simulink model "RoboticFish_NGC"  (R2023b)
settings: Solver=ode4  StartTime=0.0  StopTime=89  FixedStep=0.00025  RelTol=1e-3  EnableMultiTasking=on
undefined symbols (not defined in the file): Ref, uCMD
libraries: sharedutil x11, slpidlib x8, dspsigops x2, matrix_library x1, SignalEditorBlockLib x1, vrlib x1
(part 2 of 3)

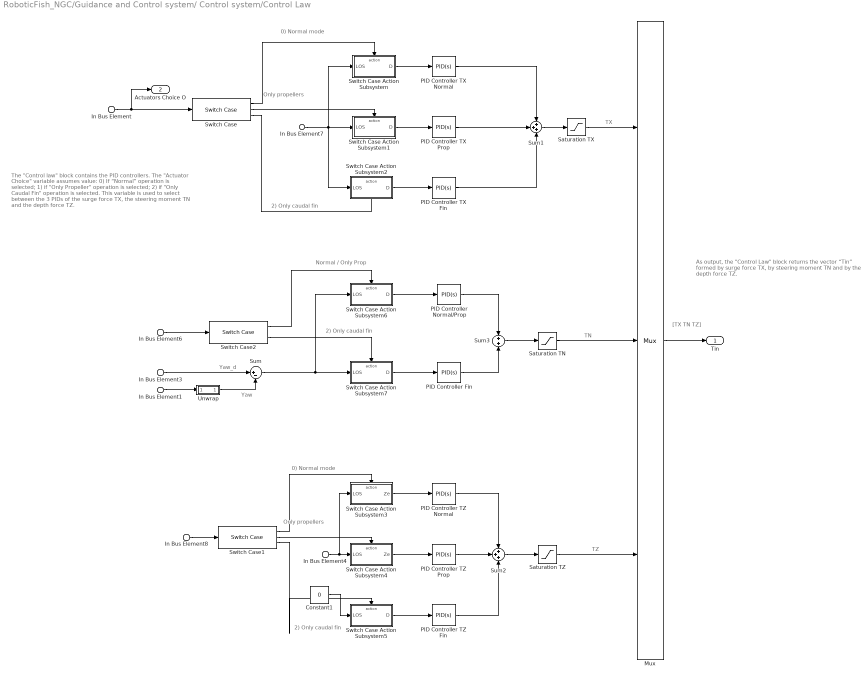
== system RoboticFish_NGC/Guidance and Control system/ Control system/Control Law ==
  note: Normal / Only Prop
  note: 2) Only caudal fin
  note: As output, the "Control Law" block returns the vector “Tin” formed by surge force TX, by steering moment TN and by the depth force TZ.
  note: The "Control law" block contains the PID controllers.
      | The "Actuator Choice" variable assumes value:
      | 0) If “Normal” operation is selected;
      | 1) if "Only Propeller" operation is selected;
      | 2) if "Only Caudal Fin" operation is selected.
      | This variable is used to select between the 3 PIDs of the surge force TX, the steering moment TN and the depth force TZ.
  note: [TX TN TZ]
  note: TZ
  note: TN
  note: TX
  note: 2) Only caudal fin
  note: Only propellers
  note: 0) Normal mode
  note: 0) Normal mode
  note: 2) Only caudal fin
  note: Only propellers
  note: Yaw
  note: Yaw_d
  In Bus Element7 : Inport  PortName=LOS  Element=D
  In Bus Element4 : Inport  PortName=LOS  Element=Ze
  In Bus Element3 : Inport  PortName=LOS  Element=Yaw_d
  In Bus Element : Inport  Port=2  PortName=P  Element=Actuators Choice
  In Bus Element8 : Inport  Port=2  PortName=P  Element=Actuators Choice
  In Bus Element6 : Inport  Port=2  PortName=P  Element=Actuators Choice
  In Bus Element1 : Inport  Port=3  PortName=Estimate States  Element=Position.Yaw
  Constant1 : Constant  Value=0
  Mux : Mux  Inputs=3
  PID Controller Fin : slpidlib/PID Controller  Controller=PID  Form=Parallel  TimeDomain=Continuous-time  UseExternalTs=off  SampleTime=-1  IntegratorMethod=Forward Euler  FilterMethod=Forward Euler  ControllerParametersSource=internal  P=0.1  I=0  UseKiTs=off  D=0.01  N=100  UseFilter=on  TunerSelectOption=Transfer Function Based (PID Tuner App)  InitialConditionSource=internal  InitialConditionForIntegrator=0  InitialConditionForFilter=0  DifferentiatorICPrevScaledInput=0  ExternalReset=none  TrackingMode=off  Kt=1  LimitOutput=off  SatLimitsSource=internal  UpperSaturationLimit=inf  LowerSaturationLimit=-inf  LinearizeAsGain=on  AntiWindupMode=none  Kb=1  LimitIntegrator=off  UpperIntegratorSaturationLimit=inf  LowerIntegratorSaturationLimit=-inf  POutMin=[]  POutMax=[]  IOutMin=[]  IOutMax=[]  DOutMin=[]  DOutMax=[]  NOutMin=[]  NOutMax=[]  SumOutMin=[]  SumOutMax=[]  SaturationOutMin=[]  SaturationOutMax=[]  PParamMin=[]  PParamMax=[]  IParamMin=[]  IParamMax=[]  DParamMin=[]  DParamMax=[]  NParamMin=[]  NParamMax=[]  KbParamMin=[]  KbParamMax=[]  KtParamMin=[]  KtParamMax=[]  KbOutMin=[]  KbOutMax=[]  KtOutMin=[]  KtOutMax=[]  IntegratorOutMin=[]  IntegratorOutMax=[]  FilterOutMin=[]  FilterOutMax=[]  SumI1OutMin=[]  SumI1OutMax=[]  SumI2OutMin=[]  SumI2OutMax=[]  SumI3OutMin=[]  SumI3OutMax=[]  SumI4OutMin=[]  SumI4OutMax=[]  SumDOutMin=[]  SumDOutMax=[]  DifferentiatorOutMin=[]  DifferentiatorOutMax=[]  FilterDiffOutCoefMin=[]  FilterDiffOutCoefMax=[]  ReciprocalOutMin=[]  ReciprocalOutMax=[]  SumDenOutMin=[]  SumDenOutMax=[]  SumNumOutMin=[]  SumNumOutMax=[]  DivideOutMin=[]  DivideOutMax=[]  UdiffTsProdOutMin=[]  UdiffTsProdOutMax=[]  NTsProdOutMin=[]  NTsProdOutMax=[]  UintegralTsProdOutMin=[]  UintegralTsProdOutMax=[]  UngainTsProdOutMin=[]  UngainTsProdOutMax=[]  ClampingZeroOutDataTypeStr=Inherit: Inherit via back propagation  ClampingZeroOutMin=[]  ClampingZeroOutMax=[]  FilterDenConstantOutDataTypeStr=Inherit: Inherit via back propagation  FilterDenConstantOutMin=[]  FilterDenConstantOutMax=[]  PCopyOutDataTypeStr=Inherit: Inherit via back propagation  PCopyOutMin=[]  PCopyOutMax=[]  NCopyOutDataTypeStr=Inherit: Inherit via back propagation  NCopyOutMin=[]  NCopyOutMax=[]  IntegratorContinuousStateAttributes=''  IntegratorStateMustResolveToSignalObject=off  IntegratorRTWStateStorageClass=Auto  FilterContinuousStateAttributes=''  FilterStateMustResolveToSignalObject=off  FilterRTWStateStorageClass=Auto  ParallelPVariant=InternalParameters  IdealPVariant=Disabled  IVariant=InternalParameters  DVariant=InternalParameters  IntegratorVariant=Continuous  SatVariant=Disabled  AWVariant=Passthrough  PCopyVariant=Disabled  TRVariant=Disabled  FdbkBlocksVariant=Forward  IdealPFdbkVariant=Disabled  SatFdbkVariant=Disabled  DerivativeFilterVariant=ContFilter  NVariant=InternalParameters  NCopyVariant=Disabled  FilterICVariant=InternalICsFilter  IntegratorICVariant=InternalICs  ExternalResetVariant=Disabled  TRSumVariant=Passthrough  SumFdbkVariant=Disabled  SumVariant=Sum_PID  TsampFilterVariant=InternalTs  TsampNgainVariant=Passthrough  TsampIntegralVariant=Disabled_SignalSpec  ExternalSaturationOutDataTypeStr=Inherit: Same as second input
  PID Controller Normal/Prop : slpidlib/PID Controller  Controller=PID  Form=Parallel  TimeDomain=Continuous-time  UseExternalTs=off  SampleTime=-1  IntegratorMethod=Forward Euler  FilterMethod=Forward Euler  ControllerParametersSource=internal  P=2  I=0  UseKiTs=off  D=1  N=100  UseFilter=on  TunerSelectOption=Transfer Function Based (PID Tuner App)  InitialConditionSource=internal  InitialConditionForIntegrator=0  InitialConditionForFilter=0  DifferentiatorICPrevScaledInput=0  ExternalReset=none  TrackingMode=off  Kt=1  LimitOutput=off  SatLimitsSource=internal  UpperSaturationLimit=inf  LowerSaturationLimit=-inf  LinearizeAsGain=on  AntiWindupMode=none  Kb=1  LimitIntegrator=off  UpperIntegratorSaturationLimit=inf  LowerIntegratorSaturationLimit=-inf  POutMin=[]  POutMax=[]  IOutMin=[]  IOutMax=[]  DOutMin=[]  DOutMax=[]  NOutMin=[]  NOutMax=[]  SumOutMin=[]  SumOutMax=[]  SaturationOutMin=[]  SaturationOutMax=[]  PParamMin=[]  PParamMax=[]  IParamMin=[]  IParamMax=[]  DParamMin=[]  DParamMax=[]  NParamMin=[]  NParamMax=[]  KbParamMin=[]  KbParamMax=[]  KtParamMin=[]  KtParamMax=[]  KbOutMin=[]  KbOutMax=[]  KtOutMin=[]  KtOutMax=[]  IntegratorOutMin=[]  IntegratorOutMax=[]  FilterOutMin=[]  FilterOutMax=[]  SumI1OutMin=[]  SumI1OutMax=[]  SumI2OutMin=[]  SumI2OutMax=[]  SumI3OutMin=[]  SumI3OutMax=[]  SumI4OutMin=[]  SumI4OutMax=[]  SumDOutMin=[]  SumDOutMax=[]  DifferentiatorOutMin=[]  DifferentiatorOutMax=[]  FilterDiffOutCoefMin=[]  FilterDiffOutCoefMax=[]  ReciprocalOutMin=[]  ReciprocalOutMax=[]  SumDenOutMin=[]  SumDenOutMax=[]  SumNumOutMin=[]  SumNumOutMax=[]  DivideOutMin=[]  DivideOutMax=[]  UdiffTsProdOutMin=[]  UdiffTsProdOutMax=[]  NTsProdOutMin=[]  NTsProdOutMax=[]  UintegralTsProdOutMin=[]  UintegralTsProdOutMax=[]  UngainTsProdOutMin=[]  UngainTsProdOutMax=[]  ClampingZeroOutDataTypeStr=Inherit: Inherit via back propagation  ClampingZeroOutMin=[]  ClampingZeroOutMax=[]  FilterDenConstantOutDataTypeStr=Inherit: Inherit via back propagation  FilterDenConstantOutMin=[]  FilterDenConstantOutMax=[]  PCopyOutDataTypeStr=Inherit: Inherit via back propagation  PCopyOutMin=[]  PCopyOutMax=[]  NCopyOutDataTypeStr=Inherit: Inherit via back propagation  NCopyOutMin=[]  NCopyOutMax=[]  IntegratorContinuousStateAttributes=''  IntegratorStateMustResolveToSignalObject=off  IntegratorRTWStateStorageClass=Auto  FilterContinuousStateAttributes=''  FilterStateMustResolveToSignalObject=off  FilterRTWStateStorageClass=Auto  ParallelPVariant=InternalParameters  IdealPVariant=Disabled  IVariant=InternalParameters  DVariant=InternalParameters  IntegratorVariant=Continuous  SatVariant=Disabled  AWVariant=Passthrough  PCopyVariant=Disabled  TRVariant=Disabled  FdbkBlocksVariant=Forward  IdealPFdbkVariant=Disabled  SatFdbkVariant=Disabled  DerivativeFilterVariant=ContFilter  NVariant=InternalParameters  NCopyVariant=Disabled  FilterICVariant=InternalICsFilter  IntegratorICVariant=InternalICs  ExternalResetVariant=Disabled  TRSumVariant=Passthrough  SumFdbkVariant=Disabled  SumVariant=Sum_PID  TsampFilterVariant=InternalTs  TsampNgainVariant=Passthrough  TsampIntegralVariant=Disabled_SignalSpec  ExternalSaturationOutDataTypeStr=Inherit: Same as second input
  PID Controller TX Fin : slpidlib/PID Controller  Controller=PID  Form=Parallel  TimeDomain=Continuous-time  UseExternalTs=off  SampleTime=-1  IntegratorMethod=Forward Euler  FilterMethod=Forward Euler  ControllerParametersSource=internal  P=1  I=0  UseKiTs=off  D=0  N=100  UseFilter=on  TunerSelectOption=Transfer Function Based (PID Tuner App)  InitialConditionSource=internal  InitialConditionForIntegrator=0  InitialConditionForFilter=0  DifferentiatorICPrevScaledInput=0  ExternalReset=none  TrackingMode=off  Kt=1  LimitOutput=off  SatLimitsSource=internal  UpperSaturationLimit=inf  LowerSaturationLimit=-inf  LinearizeAsGain=on  AntiWindupMode=none  Kb=1  LimitIntegrator=off  UpperIntegratorSaturationLimit=inf  LowerIntegratorSaturationLimit=-inf  POutMin=[]  POutMax=[]  IOutMin=[]  IOutMax=[]  DOutMin=[]  DOutMax=[]  NOutMin=[]  NOutMax=[]  SumOutMin=[]  SumOutMax=[]  SaturationOutMin=[]  SaturationOutMax=[]  PParamMin=[]  PParamMax=[]  IParamMin=[]  IParamMax=[]  DParamMin=[]  DParamMax=[]  NParamMin=[]  NParamMax=[]  KbParamMin=[]  KbParamMax=[]  KtParamMin=[]  KtParamMax=[]  KbOutMin=[]  KbOutMax=[]  KtOutMin=[]  KtOutMax=[]  IntegratorOutMin=[]  IntegratorOutMax=[]  FilterOutMin=[]  FilterOutMax=[]  SumI1OutMin=[]  SumI1OutMax=[]  SumI2OutMin=[]  SumI2OutMax=[]  SumI3OutMin=[]  SumI3OutMax=[]  SumI4OutMin=[]  SumI4OutMax=[]  SumDOutMin=[]  SumDOutMax=[]  DifferentiatorOutMin=[]  DifferentiatorOutMax=[]  FilterDiffOutCoefMin=[]  FilterDiffOutCoefMax=[]  ReciprocalOutMin=[]  ReciprocalOutMax=[]  SumDenOutMin=[]  SumDenOutMax=[]  SumNumOutMin=[]  SumNumOutMax=[]  DivideOutMin=[]  DivideOutMax=[]  UdiffTsProdOutMin=[]  UdiffTsProdOutMax=[]  NTsProdOutMin=[]  NTsProdOutMax=[]  UintegralTsProdOutMin=[]  UintegralTsProdOutMax=[]  UngainTsProdOutMin=[]  UngainTsProdOutMax=[]  ClampingZeroOutDataTypeStr=Inherit: Inherit via back propagation  ClampingZeroOutMin=[]  ClampingZeroOutMax=[]  FilterDenConstantOutDataTypeStr=Inherit: Inherit via back propagation  FilterDenConstantOutMin=[]  FilterDenConstantOutMax=[]  PCopyOutDataTypeStr=Inherit: Inherit via back propagation  PCopyOutMin=[]  PCopyOutMax=[]  NCopyOutDataTypeStr=Inherit: Inherit via back propagation  NCopyOutMin=[]  NCopyOutMax=[]  IntegratorContinuousStateAttributes=''  IntegratorStateMustResolveToSignalObject=off  IntegratorRTWStateStorageClass=Auto  FilterContinuousStateAttributes=''  FilterStateMustResolveToSignalObject=off  FilterRTWStateStorageClass=Auto  ParallelPVariant=InternalParameters  IdealPVariant=Disabled  IVariant=InternalParameters  DVariant=InternalParameters  IntegratorVariant=Continuous  SatVariant=Disabled  AWVariant=Passthrough  PCopyVariant=Disabled  TRVariant=Disabled  FdbkBlocksVariant=Forward  IdealPFdbkVariant=Disabled  SatFdbkVariant=Disabled  DerivativeFilterVariant=ContFilter  NVariant=InternalParameters  NCopyVariant=Disabled  FilterICVariant=InternalICsFilter  IntegratorICVariant=InternalICs  ExternalResetVariant=Disabled  TRSumVariant=Passthrough  SumFdbkVariant=Disabled  SumVariant=Sum_PID  TsampFilterVariant=InternalTs  TsampNgainVariant=Passthrough  TsampIntegralVariant=Disabled_SignalSpec  ExternalSaturationOutDataTypeStr=Inherit: Same as second input
  PID Controller TX Normal : slpidlib/PID Controller  Controller=PID  Form=Parallel  TimeDomain=Continuous-time  UseExternalTs=off  SampleTime=-1  IntegratorMethod=Forward Euler  FilterMethod=Forward Euler  ControllerParametersSource=internal  P=1  I=0  UseKiTs=off  D=0.2695  N=100  UseFilter=on  TunerSelectOption=Transfer Function Based (PID Tuner App)  InitialConditionSource=internal  InitialConditionForIntegrator=0  InitialConditionForFilter=0  DifferentiatorICPrevScaledInput=0  ExternalReset=none  TrackingMode=off  Kt=1  LimitOutput=off  SatLimitsSource=internal  UpperSaturationLimit=inf  LowerSaturationLimit=-inf  LinearizeAsGain=on  AntiWindupMode=none  Kb=1  LimitIntegrator=off  UpperIntegratorSaturationLimit=inf  LowerIntegratorSaturationLimit=-inf  POutMin=[]  POutMax=[]  IOutMin=[]  IOutMax=[]  DOutMin=[]  DOutMax=[]  NOutMin=[]  NOutMax=[]  SumOutMin=[]  SumOutMax=[]  SaturationOutMin=[]  SaturationOutMax=[]  PParamMin=[]  PParamMax=[]  IParamMin=[]  IParamMax=[]  DParamMin=[]  DParamMax=[]  NParamMin=[]  NParamMax=[]  KbParamMin=[]  KbParamMax=[]  KtParamMin=[]  KtParamMax=[]  KbOutMin=[]  KbOutMax=[]  KtOutMin=[]  KtOutMax=[]  IntegratorOutMin=[]  IntegratorOutMax=[]  FilterOutMin=[]  FilterOutMax=[]  SumI1OutMin=[]  SumI1OutMax=[]  SumI2OutMin=[]  SumI2OutMax=[]  SumI3OutMin=[]  SumI3OutMax=[]  SumI4OutMin=[]  SumI4OutMax=[]  SumDOutMin=[]  SumDOutMax=[]  DifferentiatorOutMin=[]  DifferentiatorOutMax=[]  FilterDiffOutCoefMin=[]  FilterDiffOutCoefMax=[]  ReciprocalOutMin=[]  ReciprocalOutMax=[]  SumDenOutMin=[]  SumDenOutMax=[]  SumNumOutMin=[]  SumNumOutMax=[]  DivideOutMin=[]  DivideOutMax=[]  UdiffTsProdOutMin=[]  UdiffTsProdOutMax=[]  NTsProdOutMin=[]  NTsProdOutMax=[]  UintegralTsProdOutMin=[]  UintegralTsProdOutMax=[]  UngainTsProdOutMin=[]  UngainTsProdOutMax=[]  ClampingZeroOutDataTypeStr=Inherit: Inherit via back propagation  ClampingZeroOutMin=[]  ClampingZeroOutMax=[]  FilterDenConstantOutDataTypeStr=Inherit: Inherit via back propagation  FilterDenConstantOutMin=[]  FilterDenConstantOutMax=[]  PCopyOutDataTypeStr=Inherit: Inherit via back propagation  PCopyOutMin=[]  PCopyOutMax=[]  NCopyOutDataTypeStr=Inherit: Inherit via back propagation  NCopyOutMin=[]  NCopyOutMax=[]  IntegratorContinuousStateAttributes=''  IntegratorStateMustResolveToSignalObject=off  IntegratorRTWStateStorageClass=Auto  FilterContinuousStateAttributes=''  FilterStateMustResolveToSignalObject=off  FilterRTWStateStorageClass=Auto  ParallelPVariant=InternalParameters  IdealPVariant=Disabled  IVariant=InternalParameters  DVariant=InternalParameters  IntegratorVariant=Continuous  SatVariant=Disabled  AWVariant=Passthrough  PCopyVariant=Disabled  TRVariant=Disabled  FdbkBlocksVariant=Forward  IdealPFdbkVariant=Disabled  SatFdbkVariant=Disabled  DerivativeFilterVariant=ContFilter  NVariant=InternalParameters  NCopyVariant=Disabled  FilterICVariant=InternalICsFilter  IntegratorICVariant=InternalICs  ExternalResetVariant=Disabled  TRSumVariant=Passthrough  SumFdbkVariant=Disabled  SumVariant=Sum_PID  TsampFilterVariant=InternalTs  TsampNgainVariant=Passthrough  TsampIntegralVariant=Disabled_SignalSpec  ExternalSaturationOutDataTypeStr=Inherit: Same as second input
  PID Controller TX Prop : slpidlib/PID Controller  Controller=PID  Form=Parallel  TimeDomain=Continuous-time  UseExternalTs=off  SampleTime=-1  IntegratorMethod=Forward Euler  FilterMethod=Forward Euler  ControllerParametersSource=internal  P=1  I=0  UseKiTs=off  D=1.2  N=100  UseFilter=on  TunerSelectOption=Frequency Response Based  InitialConditionSource=internal  InitialConditionForIntegrator=0  InitialConditionForFilter=0  DifferentiatorICPrevScaledInput=0  ExternalReset=none  TrackingMode=off  Kt=1  LimitOutput=off  SatLimitsSource=internal  UpperSaturationLimit=inf  LowerSaturationLimit=-inf  LinearizeAsGain=on  AntiWindupMode=none  Kb=1  LimitIntegrator=off  UpperIntegratorSaturationLimit=inf  LowerIntegratorSaturationLimit=-inf  POutMin=[]  POutMax=[]  IOutMin=[]  IOutMax=[]  DOutMin=[]  DOutMax=[]  NOutMin=[]  NOutMax=[]  SumOutMin=[]  SumOutMax=[]  SaturationOutMin=[]  SaturationOutMax=[]  PParamMin=[]  PParamMax=[]  IParamMin=[]  IParamMax=[]  DParamMin=[]  DParamMax=[]  NParamMin=[]  NParamMax=[]  KbParamMin=[]  KbParamMax=[]  KtParamMin=[]  KtParamMax=[]  KbOutMin=[]  KbOutMax=[]  KtOutMin=[]  KtOutMax=[]  IntegratorOutMin=[]  IntegratorOutMax=[]  FilterOutMin=[]  FilterOutMax=[]  SumI1OutMin=[]  SumI1OutMax=[]  SumI2OutMin=[]  SumI2OutMax=[]  SumI3OutMin=[]  SumI3OutMax=[]  SumI4OutMin=[]  SumI4OutMax=[]  SumDOutMin=[]  SumDOutMax=[]  DifferentiatorOutMin=[]  DifferentiatorOutMax=[]  FilterDiffOutCoefMin=[]  FilterDiffOutCoefMax=[]  ReciprocalOutMin=[]  ReciprocalOutMax=[]  SumDenOutMin=[]  SumDenOutMax=[]  SumNumOutMin=[]  SumNumOutMax=[]  DivideOutMin=[]  DivideOutMax=[]  UdiffTsProdOutMin=[]  UdiffTsProdOutMax=[]  NTsProdOutMin=[]  NTsProdOutMax=[]  UintegralTsProdOutMin=[]  UintegralTsProdOutMax=[]  UngainTsProdOutMin=[]  UngainTsProdOutMax=[]  ClampingZeroOutDataTypeStr=Inherit: Inherit via back propagation  ClampingZeroOutMin=[]  ClampingZeroOutMax=[]  FilterDenConstantOutDataTypeStr=Inherit: Inherit via back propagation  FilterDenConstantOutMin=[]  FilterDenConstantOutMax=[]  PCopyOutDataTypeStr=Inherit: Inherit via back propagation  PCopyOutMin=[]  PCopyOutMax=[]  NCopyOutDataTypeStr=Inherit: Inherit via back propagation  NCopyOutMin=[]  NCopyOutMax=[]  IntegratorContinuousStateAttributes=''  IntegratorStateMustResolveToSignalObject=off  IntegratorRTWStateStorageClass=Auto  FilterContinuousStateAttributes=''  FilterStateMustResolveToSignalObject=off  FilterRTWStateStorageClass=Auto  ParallelPVariant=InternalParameters  IdealPVariant=Disabled  IVariant=InternalParameters  DVariant=InternalParameters  IntegratorVariant=Continuous  SatVariant=Disabled  AWVariant=Passthrough  PCopyVariant=Disabled  TRVariant=Disabled  FdbkBlocksVariant=Forward  IdealPFdbkVariant=Disabled  SatFdbkVariant=Disabled  DerivativeFilterVariant=ContFilter  NVariant=InternalParameters  NCopyVariant=Disabled  FilterICVariant=InternalICsFilter  IntegratorICVariant=InternalICs  ExternalResetVariant=Disabled  TRSumVariant=Passthrough  SumFdbkVariant=Disabled  SumVariant=Sum_PID  TsampFilterVariant=InternalTs  TsampNgainVariant=Passthrough  TsampIntegralVariant=Disabled_SignalSpec  ExternalSaturationOutDataTypeStr=Inherit: Same as second input
  PID Controller TZ Fin : slpidlib/PID Controller  Controller=PID  Form=Parallel  TimeDomain=Continuous-time  UseExternalTs=off  SampleTime=-1  IntegratorMethod=Forward Euler  FilterMethod=Forward Euler  ControllerParametersSource=internal  P=0.6  I=0  UseKiTs=off  D=0.6  N=100  UseFilter=on  TunerSelectOption=Transfer Function Based (PID Tuner App)  InitialConditionSource=internal  InitialConditionForIntegrator=0  InitialConditionForFilter=0  DifferentiatorICPrevScaledInput=0  ExternalReset=none  TrackingMode=off  Kt=1  LimitOutput=off  SatLimitsSource=internal  UpperSaturationLimit=inf  LowerSaturationLimit=-inf  LinearizeAsGain=on  AntiWindupMode=none  Kb=1  LimitIntegrator=off  UpperIntegratorSaturationLimit=inf  LowerIntegratorSaturationLimit=-inf  POutMin=[]  POutMax=[]  IOutMin=[]  IOutMax=[]  DOutMin=[]  DOutMax=[]  NOutMin=[]  NOutMax=[]  SumOutMin=[]  SumOutMax=[]  SaturationOutMin=[]  SaturationOutMax=[]  PParamMin=[]  PParamMax=[]  IParamMin=[]  IParamMax=[]  DParamMin=[]  DParamMax=[]  NParamMin=[]  NParamMax=[]  KbParamMin=[]  KbParamMax=[]  KtParamMin=[]  KtParamMax=[]  KbOutMin=[]  KbOutMax=[]  KtOutMin=[]  KtOutMax=[]  IntegratorOutMin=[]  IntegratorOutMax=[]  FilterOutMin=[]  FilterOutMax=[]  SumI1OutMin=[]  SumI1OutMax=[]  SumI2OutMin=[]  SumI2OutMax=[]  SumI3OutMin=[]  SumI3OutMax=[]  SumI4OutMin=[]  SumI4OutMax=[]  SumDOutMin=[]  SumDOutMax=[]  DifferentiatorOutMin=[]  DifferentiatorOutMax=[]  FilterDiffOutCoefMin=[]  FilterDiffOutCoefMax=[]  ReciprocalOutMin=[]  ReciprocalOutMax=[]  SumDenOutMin=[]  SumDenOutMax=[]  SumNumOutMin=[]  SumNumOutMax=[]  DivideOutMin=[]  DivideOutMax=[]  UdiffTsProdOutMin=[]  UdiffTsProdOutMax=[]  NTsProdOutMin=[]  NTsProdOutMax=[]  UintegralTsProdOutMin=[]  UintegralTsProdOutMax=[]  UngainTsProdOutMin=[]  UngainTsProdOutMax=[]  ClampingZeroOutDataTypeStr=Inherit: Inherit via back propagation  ClampingZeroOutMin=[]  ClampingZeroOutMax=[]  FilterDenConstantOutDataTypeStr=Inherit: Inherit via back propagation  FilterDenConstantOutMin=[]  FilterDenConstantOutMax=[]  PCopyOutDataTypeStr=Inherit: Inherit via back propagation  PCopyOutMin=[]  PCopyOutMax=[]  NCopyOutDataTypeStr=Inherit: Inherit via back propagation  NCopyOutMin=[]  NCopyOutMax=[]  IntegratorContinuousStateAttributes=''  IntegratorStateMustResolveToSignalObject=off  IntegratorRTWStateStorageClass=Auto  FilterContinuousStateAttributes=''  FilterStateMustResolveToSignalObject=off  FilterRTWStateStorageClass=Auto  ParallelPVariant=InternalParameters  IdealPVariant=Disabled  IVariant=InternalParameters  DVariant=InternalParameters  IntegratorVariant=Continuous  SatVariant=Disabled  AWVariant=Passthrough  PCopyVariant=Disabled  TRVariant=Disabled  FdbkBlocksVariant=Forward  IdealPFdbkVariant=Disabled  SatFdbkVariant=Disabled  DerivativeFilterVariant=ContFilter  NVariant=InternalParameters  NCopyVariant=Disabled  FilterICVariant=InternalICsFilter  IntegratorICVariant=InternalICs  ExternalResetVariant=Disabled  TRSumVariant=Passthrough  SumFdbkVariant=Disabled  SumVariant=Sum_PID  TsampFilterVariant=InternalTs  TsampNgainVariant=Passthrough  TsampIntegralVariant=Disabled_SignalSpec  ExternalSaturationOutDataTypeStr=Inherit: Same as second input
  PID Controller TZ Normal : slpidlib/PID Controller  Controller=PID  Form=Parallel  TimeDomain=Continuous-time  UseExternalTs=off  SampleTime=-1  IntegratorMethod=Forward Euler  FilterMethod=Forward Euler  ControllerParametersSource=internal  P=0.6  I=0  UseKiTs=off  D=0.6  N=100  UseFilter=on  TunerSelectOption=Transfer Function Based (PID Tuner App)  InitialConditionSource=internal  InitialConditionForIntegrator=0  InitialConditionForFilter=0  DifferentiatorICPrevScaledInput=0  ExternalReset=none  TrackingMode=off  Kt=1  LimitOutput=off  SatLimitsSource=internal  UpperSaturationLimit=inf  LowerSaturationLimit=-inf  LinearizeAsGain=on  AntiWindupMode=none  Kb=1  LimitIntegrator=off  UpperIntegratorSaturationLimit=inf  LowerIntegratorSaturationLimit=-inf  POutMin=[]  POutMax=[]  IOutMin=[]  IOutMax=[]  DOutMin=[]  DOutMax=[]  NOutMin=[]  NOutMax=[]  SumOutMin=[]  SumOutMax=[]  SaturationOutMin=[]  SaturationOutMax=[]  PParamMin=[]  PParamMax=[]  IParamMin=[]  IParamMax=[]  DParamMin=[]  DParamMax=[]  NParamMin=[]  NParamMax=[]  KbParamMin=[]  KbParamMax=[]  KtParamMin=[]  KtParamMax=[]  KbOutMin=[]  KbOutMax=[]  KtOutMin=[]  KtOutMax=[]  IntegratorOutMin=[]  IntegratorOutMax=[]  FilterOutMin=[]  FilterOutMax=[]  SumI1OutMin=[]  SumI1OutMax=[]  SumI2OutMin=[]  SumI2OutMax=[]  SumI3OutMin=[]  SumI3OutMax=[]  SumI4OutMin=[]  SumI4OutMax=[]  SumDOutMin=[]  SumDOutMax=[]  DifferentiatorOutMin=[]  DifferentiatorOutMax=[]  FilterDiffOutCoefMin=[]  FilterDiffOutCoefMax=[]  ReciprocalOutMin=[]  ReciprocalOutMax=[]  SumDenOutMin=[]  SumDenOutMax=[]  SumNumOutMin=[]  SumNumOutMax=[]  DivideOutMin=[]  DivideOutMax=[]  UdiffTsProdOutMin=[]  UdiffTsProdOutMax=[]  NTsProdOutMin=[]  NTsProdOutMax=[]  UintegralTsProdOutMin=[]  UintegralTsProdOutMax=[]  UngainTsProdOutMin=[]  UngainTsProdOutMax=[]  ClampingZeroOutDataTypeStr=Inherit: Inherit via back propagation  ClampingZeroOutMin=[]  ClampingZeroOutMax=[]  FilterDenConstantOutDataTypeStr=Inherit: Inherit via back propagation  FilterDenConstantOutMin=[]  FilterDenConstantOutMax=[]  PCopyOutDataTypeStr=Inherit: Inherit via back propagation  PCopyOutMin=[]  PCopyOutMax=[]  NCopyOutDataTypeStr=Inherit: Inherit via back propagation  NCopyOutMin=[]  NCopyOutMax=[]  IntegratorContinuousStateAttributes=''  IntegratorStateMustResolveToSignalObject=off  IntegratorRTWStateStorageClass=Auto  FilterContinuousStateAttributes=''  FilterStateMustResolveToSignalObject=off  FilterRTWStateStorageClass=Auto  ParallelPVariant=InternalParameters  IdealPVariant=Disabled  IVariant=InternalParameters  DVariant=InternalParameters  IntegratorVariant=Continuous  SatVariant=Disabled  AWVariant=Passthrough  PCopyVariant=Disabled  TRVariant=Disabled  FdbkBlocksVariant=Forward  IdealPFdbkVariant=Disabled  SatFdbkVariant=Disabled  DerivativeFilterVariant=ContFilter  NVariant=InternalParameters  NCopyVariant=Disabled  FilterICVariant=InternalICsFilter  IntegratorICVariant=InternalICs  ExternalResetVariant=Disabled  TRSumVariant=Passthrough  SumFdbkVariant=Disabled  SumVariant=Sum_PID  TsampFilterVariant=InternalTs  TsampNgainVariant=Passthrough  TsampIntegralVariant=Disabled_SignalSpec  ExternalSaturationOutDataTypeStr=Inherit: Same as second input
  PID Controller TZ Prop : slpidlib/PID Controller  Controller=PID  Form=Parallel  TimeDomain=Continuous-time  UseExternalTs=off  SampleTime=-1  IntegratorMethod=Forward Euler  FilterMethod=Forward Euler  ControllerParametersSource=internal  P=0.2  I=0  UseKiTs=off  D=0.2  N=100  UseFilter=on  TunerSelectOption=Transfer Function Based (PID Tuner App)  InitialConditionSource=internal  InitialConditionForIntegrator=0  InitialConditionForFilter=0  DifferentiatorICPrevScaledInput=0  ExternalReset=none  TrackingMode=off  Kt=1  LimitOutput=off  SatLimitsSource=internal  UpperSaturationLimit=inf  LowerSaturationLimit=-inf  LinearizeAsGain=on  AntiWindupMode=none  Kb=1  LimitIntegrator=off  UpperIntegratorSaturationLimit=inf  LowerIntegratorSaturationLimit=-inf  POutMin=[]  POutMax=[]  IOutMin=[]  IOutMax=[]  DOutMin=[]  DOutMax=[]  NOutMin=[]  NOutMax=[]  SumOutMin=[]  SumOutMax=[]  SaturationOutMin=[]  SaturationOutMax=[]  PParamMin=[]  PParamMax=[]  IParamMin=[]  IParamMax=[]  DParamMin=[]  DParamMax=[]  NParamMin=[]  NParamMax=[]  KbParamMin=[]  KbParamMax=[]  KtParamMin=[]  KtParamMax=[]  KbOutMin=[]  KbOutMax=[]  KtOutMin=[]  KtOutMax=[]  IntegratorOutMin=[]  IntegratorOutMax=[]  FilterOutMin=[]  FilterOutMax=[]  SumI1OutMin=[]  SumI1OutMax=[]  SumI2OutMin=[]  SumI2OutMax=[]  SumI3OutMin=[]  SumI3OutMax=[]  SumI4OutMin=[]  SumI4OutMax=[]  SumDOutMin=[]  SumDOutMax=[]  DifferentiatorOutMin=[]  DifferentiatorOutMax=[]  FilterDiffOutCoefMin=[]  FilterDiffOutCoefMax=[]  ReciprocalOutMin=[]  ReciprocalOutMax=[]  SumDenOutMin=[]  SumDenOutMax=[]  SumNumOutMin=[]  SumNumOutMax=[]  DivideOutMin=[]  DivideOutMax=[]  UdiffTsProdOutMin=[]  UdiffTsProdOutMax=[]  NTsProdOutMin=[]  NTsProdOutMax=[]  UintegralTsProdOutMin=[]  UintegralTsProdOutMax=[]  UngainTsProdOutMin=[]  UngainTsProdOutMax=[]  ClampingZeroOutDataTypeStr=Inherit: Inherit via back propagation  ClampingZeroOutMin=[]  ClampingZeroOutMax=[]  FilterDenConstantOutDataTypeStr=Inherit: Inherit via back propagation  FilterDenConstantOutMin=[]  FilterDenConstantOutMax=[]  PCopyOutDataTypeStr=Inherit: Inherit via back propagation  PCopyOutMin=[]  PCopyOutMax=[]  NCopyOutDataTypeStr=Inherit: Inherit via back propagation  NCopyOutMin=[]  NCopyOutMax=[]  IntegratorContinuousStateAttributes=''  IntegratorStateMustResolveToSignalObject=off  IntegratorRTWStateStorageClass=Auto  FilterContinuousStateAttributes=''  FilterStateMustResolveToSignalObject=off  FilterRTWStateStorageClass=Auto  ParallelPVariant=InternalParameters  IdealPVariant=Disabled  IVariant=InternalParameters  DVariant=InternalParameters  IntegratorVariant=Continuous  SatVariant=Disabled  AWVariant=Passthrough  PCopyVariant=Disabled  TRVariant=Disabled  FdbkBlocksVariant=Forward  IdealPFdbkVariant=Disabled  SatFdbkVariant=Disabled  DerivativeFilterVariant=ContFilter  NVariant=InternalParameters  NCopyVariant=Disabled  FilterICVariant=InternalICsFilter  IntegratorICVariant=InternalICs  ExternalResetVariant=Disabled  TRSumVariant=Passthrough  SumFdbkVariant=Disabled  SumVariant=Sum_PID  TsampFilterVariant=InternalTs  TsampNgainVariant=Passthrough  TsampIntegralVariant=Disabled_SignalSpec  ExternalSaturationOutDataTypeStr=Inherit: Same as second input
  Saturation TN : Saturate  UpperLimit=1.3090  LowerLimit=-1.3090
  Saturation TX : Saturate  UpperLimit=4  LowerLimit=0
  Saturation TZ : Saturate  UpperLimit=1  LowerLimit=-1
  Sum : Sum  Inputs=|+-
  Sum1 : Sum  Inputs=+++
  Sum2 : Sum  Inputs=+++
  Sum3 : Sum
  Switch Case : SwitchCase  CaseConditions={0,1,2}  ShowDefaultCase=off
  Switch Case Action Subsystem : Subsystem  TreatAsAtomicUnit=on
  Switch Case Action Subsystem1 : Subsystem  TreatAsAtomicUnit=on
  Switch Case Action Subsystem2 : Subsystem  TreatAsAtomicUnit=on
  Switch Case Action Subsystem3 : Subsystem  TreatAsAtomicUnit=on
  Switch Case Action Subsystem4 : Subsystem  TreatAsAtomicUnit=on
  Switch Case Action Subsystem5 : Subsystem  TreatAsAtomicUnit=on
  Switch Case Action Subsystem6 : Subsystem  TreatAsAtomicUnit=on
  Switch Case Action Subsystem7 : Subsystem  TreatAsAtomicUnit=on
  Switch Case1 : SwitchCase  CaseConditions={0,1,2}  ShowDefaultCase=off
  Switch Case2 : SwitchCase  CaseConditions={[0,1],2}  ShowDefaultCase=off
  Unwrap : Subsystem
  Tin : Outport  VectorParamsAs1DForOutWhenUnconnected=off
  Actuators Choice O : Outport  Port=2  VectorParamsAs1DForOutWhenUnconnected=off
  wires:
  In Bus Element/1 -> Switch Case/1, Actuators Choice O/1
  Switch Case/1 -> Switch Case Action Subsystem/Action
  Switch Case/2 -> Switch Case Action Subsystem1/Action
  Switch Case/3 -> Switch Case Action Subsystem2/Action
  In Bus Element7/1 -> Switch Case Action Subsystem1/1(LOS), Switch Case Action Subsystem/1(LOS), Switch Case Action Subsystem2/1(LOS)
  Switch Case Action Subsystem/1(D) -> PID Controller TX Normal/1
  Switch Case Action Subsystem1/1(D) -> PID Controller TX Prop/1
  Switch Case Action Subsystem2/1(D) -> PID Controller TX Fin/1
  PID Controller TX Prop/1 -> Sum1/2
  PID Controller TX Normal/1 -> Sum1/1
  Sum1/1 -> Saturation TX/1
  Sum2/1 -> Saturation TZ/1
  Switch Case Action Subsystem3/1(Ze) -> PID Controller TZ Normal/1
  Switch Case Action Subsystem5/1(D) -> PID Controller TZ Fin/1
  PID Controller TZ Prop/1 -> Sum2/2
  Switch Case Action Subsystem4/1(Ze) -> PID Controller TZ Prop/1
  Switch Case1/3 -> Switch Case Action Subsystem5/Action
  Switch Case1/2 -> Switch Case Action Subsystem4/Action
  Switch Case1/1 -> Switch Case Action Subsystem3/Action
  In Bus Element8/1 -> Switch Case1/1
  In Bus Element4/1 -> Switch Case Action Subsystem3/1(LOS), Switch Case Action Subsystem4/1(LOS)
  PID Controller TZ Fin/1 -> Sum2/3
  PID Controller TZ Normal/1 -> Sum2/1
  Constant1/1 -> Switch Case Action Subsystem5/1(LOS)
  Saturation TX/1 -> Mux/1
  Saturation TN/1 -> Mux/2
  Saturation TZ/1 -> Mux/3
  Mux/1 -> Tin/1
  Sum3/1 -> Saturation TN/1
  In Bus Element3/1 -> Sum/1
  In Bus Element1/1 -> Unwrap/1(yaw in)
  Unwrap/1(yaw out) -> Sum/2
  Switch Case2/1 -> Switch Case Action Subsystem6/Action
  Switch Case2/2 -> Switch Case Action Subsystem7/Action
  Switch Case Action Subsystem6/1(D) -> PID Controller Normal/Prop/1
  Switch Case Action Subsystem7/1(D) -> PID Controller Fin/1
  PID Controller Normal/Prop/1 -> Sum3/1
  PID Controller Fin/1 -> Sum3/2
  In Bus Element6/1 -> Switch Case2/1
  Sum/1 -> Switch Case Action Subsystem7/1(LOS), Switch Case Action Subsystem6/1(LOS)
  PID Controller TX Fin/1 -> Sum1/3

== system RoboticFish_NGC/Guidance and Control system/ Guidance system/Distance ==
  "[Xe Ye]" : Inport
  Demux : Demux  Outputs=2
  Plus : Sum
  Sqrt : Sqrt
  Square : Math  Operator=square  SignedPower=on
  Square1 : Math  Operator=square  SignedPower=on
  D : Outport  VectorParamsAs1DForOutWhenUnconnected=off
  wires:
  Demux/2 -> Square1/1  "Y"
  Square/1 -> Plus/1  "X^2"
  Square1/1 -> Plus/2  "Y^2"
  Plus/1 -> Sqrt/1  "X^2 + Y^2"
  Sqrt/1 -> D/1  "sqrt(X^2 + Y^2 )"
  Demux/1 -> Square/1  "X"
  "[Xe Ye]"/1 -> Demux/1

== system RoboticFish_NGC/Guidance and Control system/ Guidance system/LOS law ==
  note: To calculate the angle Yaw_d, the Unwrap Simulink block unwraps the input by adding or subtracting appropriate multiples of 𝜋 to remove phase discontinuities.
  "[Xe Ye]" : Inport
  Atan2 : Trigonometry  Operator=atan2
  Gain3 : Gain  Gain=180/pi
  Selector : Selector  InputPortWidth=2  IndexOptions=Index vector (dialog)  Indices=[2]  OutputSizes=1
  Selector3 : Selector  InputPortWidth=2  IndexOptions=Index vector (dialog)  Indices=[1]  OutputSizes=1
  "Unwrap " : dspsigops/Unwrap  tol=pi  InputProcessing=Columns as channels (frame based)  running=off
  Yaw_d : Outport  VectorParamsAs1DForOutWhenUnconnected=off
  wires:
  Selector/1 -> Atan2/1  "Ye"
  Selector3/1 -> Atan2/2  "Xe"
  "[Xe Ye]"/1 -> Selector3/1, Selector/1
  Gain3/1 -> Yaw_d/1
  Atan2/1 -> "Unwrap "/1
  "Unwrap "/1 -> Gain3/1

== system RoboticFish_NGC/Robotic-Fish Model & PropulsionSystem/Propulsion System/Horizontal Force and Moment (Tau_H) ==
  note: calcolo modulo: U=modulo(u v w)
  uHT3 : Inport
  uHT1 : Inport  Port=2
  uHT2 : Inport  Port=3
  nu_B : Inport  Port=4
  Dot Product : DotProduct  OutDataTypeStr=Inherit: Inherit via internal rule
  HT_prop : Constant  Value=HT_prop
  Matrix Multiply : Product  Multiplication=Matrix(*)
  Mux : Mux  Inputs=3
  Mux1 : Mux  Inputs=2
  Selector : Selector  InputPortWidth=6  IndexOptions=Index vector (dialog)  Indices=[1 2 3]  OutputSizes=1
  Sqrt : Sqrt
  Sum : Sum  Inputs=|++
  Tau_HT3 (Tau_Caudal_Fin) : Subsystem
  t : Clock
  Horizontal _Tau : Outport  VectorParamsAs1DForOutWhenUnconnected=off
  wires:
  uHT1/1 -> Mux1/1
  Tau_HT3 (Tau_Caudal_Fin)/1(Tau_HT3) -> Sum/1  "[Tau_surge_HT3 Tau_sway_HT3 0 0 0 Tau_yaw_HT3]"
  uHT2/1 -> Mux1/2
  Matrix Multiply/1 -> Sum/2  "[surge_HT1&HT2 0 0 0 0 yaw_HT1&HT2]"
  Mux1/1 -> Matrix Multiply/2
  HT_prop/1 -> Matrix Multiply/1
  Sum/1 -> Horizontal _Tau/1  "Tau_HT3+Tau_HT1&HT2"
  nu_B/1 -> Selector/1
  Selector/1 -> Dot Product/1, Dot Product/2
  Mux/1 -> Tau_HT3 (Tau_Caudal_Fin)/1("[U uHT3 t]")
  t/1 -> Mux/3
  Dot Product/1 -> Sqrt/1
  uHT3/1 -> Mux/2  "[f_%  Thetastr_%]"
  Sqrt/1 -> Mux/1  "U"

== system RoboticFish_NGC/Robotic-Fish Model & PropulsionSystem/Propulsion System/Subsystem ==
  D_uVT2  D_uVT3 : Inport
  uCMD : Inport  Port=2
  Bus Creator : BusCreator  Inputs=7
  Bus Selector : BusSelector  OutputSignals=D_VT2,D_VT3
  Bus Selector1 : BusSelector  OutputSignals=f_HT3,Thetastr_HT3,uHT1,uHT2,uVT1
  "ucmd " : Outport  VectorParamsAs1DForOutWhenUnconnected=off
  wires:
  D_uVT2  D_uVT3/1 -> Bus Selector/1
  uCMD/1 -> Bus Selector1/1
  Bus Selector/1 -> Bus Creator/6  "<D_VT2>"
  Bus Selector/2 -> Bus Creator/7  "<D_VT3>"
  Bus Selector1/5 -> Bus Creator/5  "<uVT1>"
  Bus Selector1/4 -> Bus Creator/4  "<uHT2>"
  Bus Selector1/3 -> Bus Creator/3  "<uHT1>"
  Bus Selector1/2 -> Bus Creator/2  "<Thetastr_HT3>"
  Bus Selector1/1 -> Bus Creator/1  "<f_HT3>"
  Bus Creator/1 -> "ucmd "/1

== system RoboticFish_NGC/Robotic-Fish Model & PropulsionSystem/Propulsion System/Vertical Force and Moment (Tau_V) ==
  note: Tau_VT2&VT3= [ 0 Ys Zs Ks Ms Ns ]
  note: Tau_VT1=[0 0 0 0 0 Fvt1]
  nu_B : Inport
  uVT1 : Inport  Port=2
  "[uVT2 uVT3]" : Inport  Port=3
  Bus Creator : BusCreator  Inputs=2
  Bus Selector : BusSelector  OutputSignals=uVT2,uVT3
  Constant : Constant  Value=VT_prop
  Matrix Multiply : Product  Multiplication=Matrix(*)
  Sum : Sum  Inputs=|++
  Tau_VT2&VT3 (Pectoral Fin) : Subsystem
  Vertical_Tau : Outport  VectorParamsAs1DForOutWhenUnconnected=off
  "[Delta_VT2 Delta_VT3]" : Outport  Port=2  VectorParamsAs1DForOutWhenUnconnected=off
  wires:
  nu_B/1 -> Tau_VT2&VT3 (Pectoral Fin)/3(nu_B)
  Constant/1 -> Matrix Multiply/1
  uVT1/1 -> Matrix Multiply/2
  Matrix Multiply/1 -> Sum/2
  Sum/1 -> Vertical_Tau/1
  Tau_VT2&VT3 (Pectoral Fin)/2(Delta_VT2) -> Bus Creator/1  "D_VT2"
  Tau_VT2&VT3 (Pectoral Fin)/3(Delta_VT3) -> Bus Creator/2  "D_VT3"
  Bus Creator/1 -> "[Delta_VT2 Delta_VT3]"/1
  Tau_VT2&VT3 (Pectoral Fin)/1("tau_VT2 & tau_VT3 ") -> Sum/1
  "[uVT2 uVT3]"/1 -> Bus Selector/1
  Bus Selector/1 -> Tau_VT2&VT3 (Pectoral Fin)/1("uVT2 ")  "<uVT2>"
  Bus Selector/2 -> Tau_VT2&VT3 (Pectoral Fin)/2(uVT3)  "<uVT3>"

== system RoboticFish_NGC/Robotic-Fish Model & PropulsionSystem/RF Dynamics and Kinematics (Attitude rappresentation: Quaternions)/6 DOF transformation ==
  note: p q r
  note: u v w
  note: e=[eta;e1;e2;e3]
  note: eta1dot
  note: eta2dot
  eta_E : Inport
  nu : Inport  Port=2
  E1(e) : Subsystem
  E2(e) : Subsystem
  Mux : Mux  Inputs=2
  Product : Product  Inputs=**  Multiplication=Matrix(*)  SaturateOnIntegerOverflow=on  OutDataTypeStr=Inherit: Same as first input
  Product1 : Product  Inputs=**  Multiplication=Matrix(*)  SaturateOnIntegerOverflow=on  OutDataTypeStr=Inherit: Same as first input
  Selector : Selector  InputPortWidth=7  IndexOptions=Index vector (dialog)  Indices=[4 5 6 7]  OutputSizes=1
  Selector1 : Selector  InputPortWidth=6  IndexOptions=Index vector (dialog)  Indices=[1 2 3]  OutputSizes=1
  Selector2 : Selector  InputPortWidth=6  IndexOptions=Index vector (dialog)  Indices=[4 5 6]  OutputSizes=1
  etadot = J(eta_E)*nu : Outport  VectorParamsAs1DForOutWhenUnconnected=off
  E1 : Outport  Port=2  VectorParamsAs1DForOutWhenUnconnected=off
  wires:
  Product1/1 -> Mux/2
  Mux/1 -> etadot = J(eta_E)*nu/1
  Product/1 -> Mux/1
  E2(e)/1(E2) -> Product1/1
  Selector2/1 -> Product1/2
  Selector1/1 -> Product/2
  nu/1 -> Selector2/1, Selector1/1
  E1(e)/1(E1) -> Product/1, E1/1
  eta_E/1 -> Selector/1
  Selector/1 -> E1(e)/1(e), E2(e)/1(e)

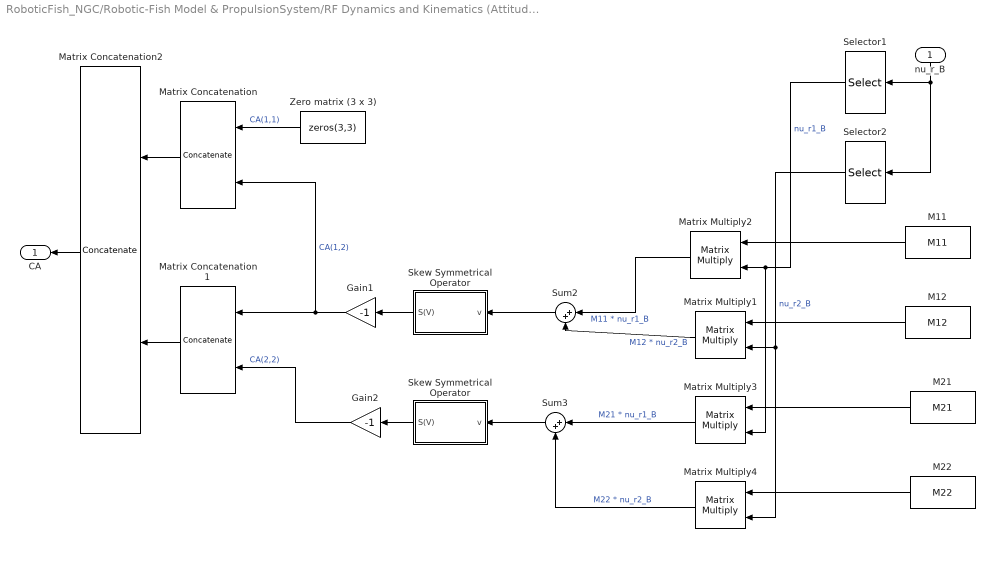
== system RoboticFish_NGC/Robotic-Fish Model & PropulsionSystem/RF Dynamics and Kinematics (Attitude rappresentation: Quaternions)/Added Mass Coriolis and centripetal matrix ==
  nu_r_B : Inport
  Gain1 : Gain  Gain=-1  SaturateOnIntegerOverflow=on  OutDataTypeStr=Inherit: Same as input  ParamDataTypeStr=Inherit: Same as input
  Gain2 : Gain  Gain=-1  SaturateOnIntegerOverflow=on  OutDataTypeStr=Inherit: Same as input  ParamDataTypeStr=Inherit: Same as input
  M11 : Constant  Value=M11
  M12 : Constant  Value=M12
  M21 : Constant  Value=M21
  M22 : Constant  Value=M22
  Matrix Concatenation : Concatenate  Mode=Multidimensional array
  Matrix Concatenation1 : Concatenate  Mode=Multidimensional array
  Matrix Concatenation2 : Concatenate  Mode=Multidimensional array  ConcatenateDimension=2
  Matrix Multiply{1..4} (4 alike) : Product  Multiplication=Matrix(*)
  Selector1 : Selector  InputPortWidth=6  IndexOptions=Index vector (dialog)  Indices=[1 2 3]  OutputSizes=1
  Selector2 : Selector  InputPortWidth=6  IndexOptions=Index vector (dialog)  Indices=[4 5 6]  OutputSizes=1
  Skew Symmetrical Operator : Subsystem
  "Skew Symmetrical Operator " : Subsystem
  Sum2 : Sum  Inputs=|++  SaturateOnIntegerOverflow=on
  Sum3 : Sum  Inputs=|++  SaturateOnIntegerOverflow=on
  Zero matrix (3 x 3) : Constant  Value=zeros(3,3)
  CA : Outport  VectorParamsAs1DForOutWhenUnconnected=off
  wires:
  Zero matrix (3 x 3)/1 -> Matrix Concatenation/1  "CA(1,1)"
  Matrix Concatenation/1 -> Matrix Concatenation2/1
  Matrix Concatenation1/1 -> Matrix Concatenation2/2
  Matrix Multiply2/1 -> Sum2/1  "M11 * nu_r1_B"
  Matrix Multiply1/1 -> Sum2/2  "M12 * nu_r2_B"
  Matrix Multiply3/1 -> Sum3/1  "M21 * nu_r1_B"
  Selector1/1 -> Matrix Multiply2/2, Matrix Multiply3/2  "nu_r1_B"
  Matrix Multiply4/1 -> Sum3/2  "M22 * nu_r2_B"
  Selector2/1 -> Matrix Multiply1/2, Matrix Multiply4/2  "nu_r2_B"
  Sum2/1 -> "Skew Symmetrical Operator "/1(v)
  Sum3/1 -> Skew Symmetrical Operator/1(v)
  "Skew Symmetrical Operator "/1(S(V)) -> Gain1/1
  Skew Symmetrical Operator/1(S(V)) -> Gain2/1
  Gain1/1 -> Matrix Concatenation1/1, Matrix Concatenation/2  "CA(1,2)"
  Gain2/1 -> Matrix Concatenation1/2  "CA(2,2)"
  nu_r_B/1 -> Selector1/1, Selector2/1
  Matrix Concatenation2/1 -> CA/1
  M11/1 -> Matrix Multiply2/1
  M12/1 -> Matrix Multiply1/1
  M21/1 -> Matrix Multiply3/1
  M22/1 -> Matrix Multiply4/1

== system RoboticFish_NGC/Robotic-Fish Model & PropulsionSystem/RF Dynamics and Kinematics (Attitude rappresentation: Quaternions)/Damping forces ==
  nu_r_B : Inport
  Abs : Abs
  Create Diagonal Matrix : matrix_library/Create Diagonal Matrix
  Linear Damping Matrix : Constant  Value=DL
  Matrix Multiply : Product  Multiplication=Matrix(*)
  Product : Product  SaturateOnIntegerOverflow=on  OutDataTypeStr=Inherit: Same as first input
  Quadratic Damping Vector : Constant  Value=dQ
  Reshape1 : Reshape  OutputDimensionality=Column vector (2-D)
  Reshape2 : Reshape  OutputDimensionality=Column vector (2-D)  OutputDimensions=[6,6]
  Sum1 : Sum  Inputs=|++  SaturateOnIntegerOverflow=on
  D * nu_B : Outport  VectorParamsAs1DForOutWhenUnconnected=off
  wires:
  Reshape2/1 -> Product/1
  Reshape1/1 -> Matrix Multiply/2, Abs/1
  nu_r_B/1 -> Reshape1/1
  Linear Damping Matrix/1 -> Sum1/1
  Create Diagonal Matrix/1 -> Sum1/2
  Product/1 -> Create Diagonal Matrix/1
  Abs/1 -> Product/2  "abs(nu_B)"
  Quadratic Damping Vector/1 -> Reshape2/1  "dQ"
  Matrix Multiply/1 -> D * nu_B/1
  Sum1/1 -> Matrix Multiply/1  "D"

== system RoboticFish_NGC/Robotic-Fish Model & PropulsionSystem/RF Dynamics and Kinematics (Attitude rappresentation: Quaternions)/Quaternion normalisation ==
  eta_E : Inport
  Mux : Mux  Inputs=2
  Product : Product  Inputs=*/  SaturateOnIntegerOverflow=on  OutDataTypeStr=Inherit: Same as first input
  Reshape : Reshape  OutputDimensionality=Column vector (2-D)
  Selector : Selector  InputPortWidth=7  IndexOptions=Index vector (dialog)  Indices=[1 2 3]  OutputSizes=1
  Selector1 : Selector  InputPortWidth=7  IndexOptions=Index vector (dialog)  Indices=[4 5 6 7]  OutputSizes=1
  norm 1x4 vector : Subsystem
  eta_E (norm) : Outport  VectorParamsAs1DForOutWhenUnconnected=off
  wires:
  eta_E/1 -> Selector1/1, Selector/1  "eta_E"
  Selector1/1 -> norm 1x4 vector/1(Inport), Product/1
  Selector/1 -> Mux/1
  Product/1 -> Mux/2
  Mux/1 -> Reshape/1
  Reshape/1 -> eta_E (norm)/1
  norm 1x4 vector/1(norm) -> Product/2

== system RoboticFish_NGC/Robotic-Fish Model & PropulsionSystem/RF Dynamics and Kinematics (Attitude rappresentation: Quaternions)/Restoring forces ==
  eta_E : Inport
  3x3 Cross Product : sharedutil/3x3 Cross Product  aMode=aMode
  3x3 Cross Product1 : sharedutil/3x3 Cross Product  aMode=aMode
  E1(e) : Subsystem
  Gain : Gain  Gain=-1  SaturateOnIntegerOverflow=on  OutDataTypeStr=Inherit: Same as input  ParamDataTypeStr=Inherit: Same as input
  Matrix Multiply : Product  Multiplication=Matrix(*)
  Matrix Multiply1 : Product  Multiplication=Matrix(*)
  Mux : Mux  Inputs=2
  Selector : Selector  InputPortWidth=7  IndexOptions=Index vector (dialog)  Indices=[4 5 6 7]  OutputSizes=1
  Sum1 : Sum  Inputs=|++  SaturateOnIntegerOverflow=on
  Sum2 : Sum  Inputs=|++  SaturateOnIntegerOverflow=on
  Transpose : Math  Operator=transpose  SignedPower=on
  fB_E : Constant  Value=[0;0;-B]
  fG_E : Constant  Value=[0;0;W]
  rB_B : Constant  Value=rB_B
  rG_B : Constant  Value=rG_B
  g(eta_E)_B : Outport  VectorParamsAs1DForOutWhenUnconnected=off
  wires:
  E1(e)/1(E1) -> Transpose/1  "E1(e)"
  Transpose/1 -> Matrix Multiply/1, Matrix Multiply1/1  "E1(e)^T"
  fG_E/1 -> Matrix Multiply/2
  fB_E/1 -> Matrix Multiply1/2
  Matrix Multiply/1 -> Sum1/1, 3x3 Cross Product/2  "fG_B"
  Matrix Multiply1/1 -> Sum1/2, 3x3 Cross Product1/2  "fB_B"
  rG_B/1 -> 3x3 Cross Product/1
  Sum1/1 -> Mux/1  "fG_B + fB_B"
  3x3 Cross Product/1 -> Sum2/1  "rG_B x fG_B"
  3x3 Cross Product1/1 -> Sum2/2  "rG_B x fG_B"
  rB_B/1 -> 3x3 Cross Product1/1
  Sum2/1 -> Mux/2
  Mux/1 -> Gain/1
  Gain/1 -> g(eta_E)_B/1
  Selector/1 -> E1(e)/1(e)  "e"
  eta_E/1 -> Selector/1  "E1(e)"

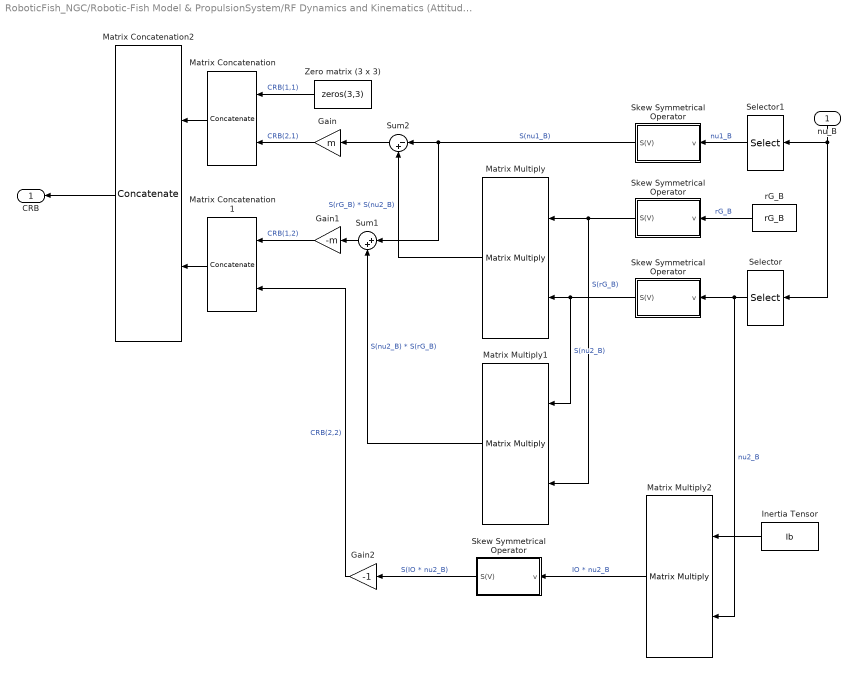
== system RoboticFish_NGC/Robotic-Fish Model & PropulsionSystem/RF Dynamics and Kinematics (Attitude rappresentation: Quaternions)/Rigid-body Coriolis and centripetal matrix ==
  nu_B : Inport
  Gain : Gain  Gain=m  SaturateOnIntegerOverflow=on  OutDataTypeStr=Inherit: Same as input  ParamDataTypeStr=Inherit: Same as input
  Gain1 : Gain  Gain=-m  SaturateOnIntegerOverflow=on  OutDataTypeStr=Inherit: Same as input  ParamDataTypeStr=Inherit: Same as input
  Gain2 : Gain  Gain=-1  SaturateOnIntegerOverflow=on  OutDataTypeStr=Inherit: Same as input  ParamDataTypeStr=Inherit: Same as input
  Inertia Tensor : Constant  Value=Ib
  Matrix Concatenation : Concatenate  Mode=Multidimensional array
  Matrix Concatenation1 : Concatenate  Mode=Multidimensional array
  Matrix Concatenation2 : Concatenate  Mode=Multidimensional array  ConcatenateDimension=2
  Matrix Multiply : Product  Multiplication=Matrix(*)
  Matrix Multiply1 : Product  Multiplication=Matrix(*)
  Matrix Multiply2 : Product  Multiplication=Matrix(*)
  Selector : Selector  InputPortWidth=6  IndexOptions=Index vector (dialog)  Indices=[4 5 6]  OutputSizes=1
  Selector1 : Selector  InputPortWidth=6  IndexOptions=Index vector (dialog)  Indices=[1 2 3]  OutputSizes=1
  "Skew Symmetrical Operator " : Subsystem
  Skew Symmetrical Operator : Subsystem
  "Skew Symmetrical Operator " : Subsystem
  "Skew Symmetrical Operator  " : Subsystem
  Sum1 : Sum  Inputs=|++  SaturateOnIntegerOverflow=on
  Sum2 : Sum  Inputs=|-+  SaturateOnIntegerOverflow=on
  Zero matrix (3 x 3) : Constant  Value=zeros(3,3)
  rG_B : Constant  Value=rG_B
  CRB : Outport  VectorParamsAs1DForOutWhenUnconnected=off
  wires:
  Gain2/1 -> Matrix Concatenation1/2  "CRB(2,2)"
  Gain/1 -> Matrix Concatenation/2  "CRB(2,1)"
  rG_B/1 -> "Skew Symmetrical Operator  "/1(v)  "rG_B"
  "Skew Symmetrical Operator "/1(S(V)) -> Gain2/1  "S(IO * nu2_B)"
  Selector1/1 -> Skew Symmetrical Operator/1(v)  "nu1_B"
  nu_B/1 -> Selector/1, Selector1/1
  Matrix Concatenation2/1 -> CRB/1
  Skew Symmetrical Operator/1(S(V)) -> Sum2/1, Sum1/1  "S(nu1_B)"
  Gain1/1 -> Matrix Concatenation1/1  "CRB(1,2)"
  Zero matrix (3 x 3)/1 -> Matrix Concatenation/1  "CRB(1,1)"
  Matrix Multiply2/1 -> "Skew Symmetrical Operator "/1(v)  "IO * nu2_B"
  Sum2/1 -> Gain/1
  Matrix Concatenation1/1 -> Matrix Concatenation2/2
  Selector/1 -> "Skew Symmetrical Operator "/1(v), Matrix Multiply2/2  "nu2_B"
  Matrix Multiply/1 -> Sum2/2  "S(rG_B) * S(nu2_B)"
  Inertia Tensor/1 -> Matrix Multiply2/1
  Matrix Concatenation/1 -> Matrix Concatenation2/1
  "Skew Symmetrical Operator "/1(S(V)) -> Matrix Multiply/2, Matrix Multiply1/1  "S(nu2_B)"
  Sum1/1 -> Gain1/1
  Matrix Multiply1/1 -> Sum1/2  "S(nu2_B) * S(rG_B)"
  "Skew Symmetrical Operator  "/1(S(V)) -> Matrix Multiply/1, Matrix Multiply1/2  "S(rG_B)"

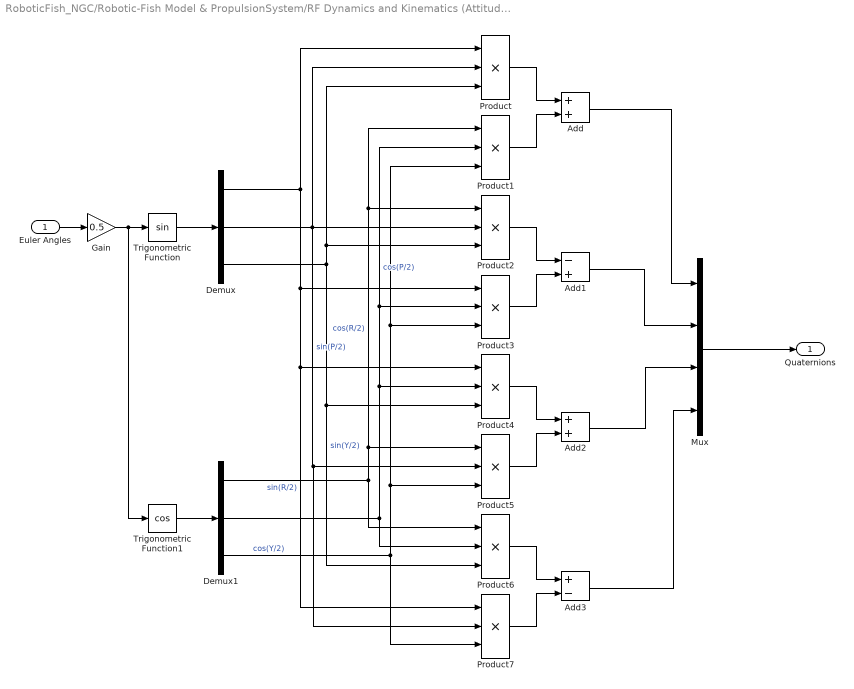
== system RoboticFish_NGC/Robotic-Fish Model & PropulsionSystem/RF Dynamics and Kinematics (Attitude rappresentation: Quaternions)/Subsystem ==
  "Euler Angles " : Inport
  Add : Sum
  Add1 : Sum  Inputs=-+
  Add2 : Sum
  Add3 : Sum  Inputs=+-
  Demux : Demux  Outputs=3
  Demux1 : Demux  Outputs=3
  Gain : Gain  Gain=0.5
  Mux : Mux
  Product{,1..7} (8 alike) : Product  Inputs=3
  Trigonometric Function : Trigonometry
  Trigonometric Function1 : Trigonometry  Operator=cos
  Quaternions : Outport  VectorParamsAs1DForOutWhenUnconnected=off
  wires:
  "Euler Angles "/1 -> Gain/1
  Gain/1 -> Trigonometric Function1/1, Trigonometric Function/1
  Trigonometric Function/1 -> Demux/1
  Demux/1 -> Product7/1, Product4/1, Product3/1, Product/1  "sin(R/2)"
  Demux/2 -> Product7/2, Product5/2, Product2/2, Product/2  "sin(P/2)"
  Demux/3 -> Product6/3, Product4/3, Product2/3, Product/3  "sin(Y/2)"
  Trigonometric Function1/1 -> Demux1/1
  Demux1/2 -> Product4/2, Product3/2, Product1/2, Product6/2  "cos(P/2)"
  Demux1/1 -> Product6/1, Product1/1, Product2/1, Product5/1  "cos(R/2)"
  Demux1/3 -> Product7/3, Product3/3, Product1/3, Product5/3  "cos(Y/2)"
  Product/1 -> Add/1
  Product1/1 -> Add/2
  Product2/1 -> Add1/1
  Product3/1 -> Add1/2
  Product4/1 -> Add2/1
  Product5/1 -> Add2/2
  Product6/1 -> Add3/1
  Product7/1 -> Add3/2
  Mux/1 -> Quaternions/1
  Add1/1 -> Mux/2
  Add/1 -> Mux/1
  Add2/1 -> Mux/3
  Add3/1 -> Mux/4

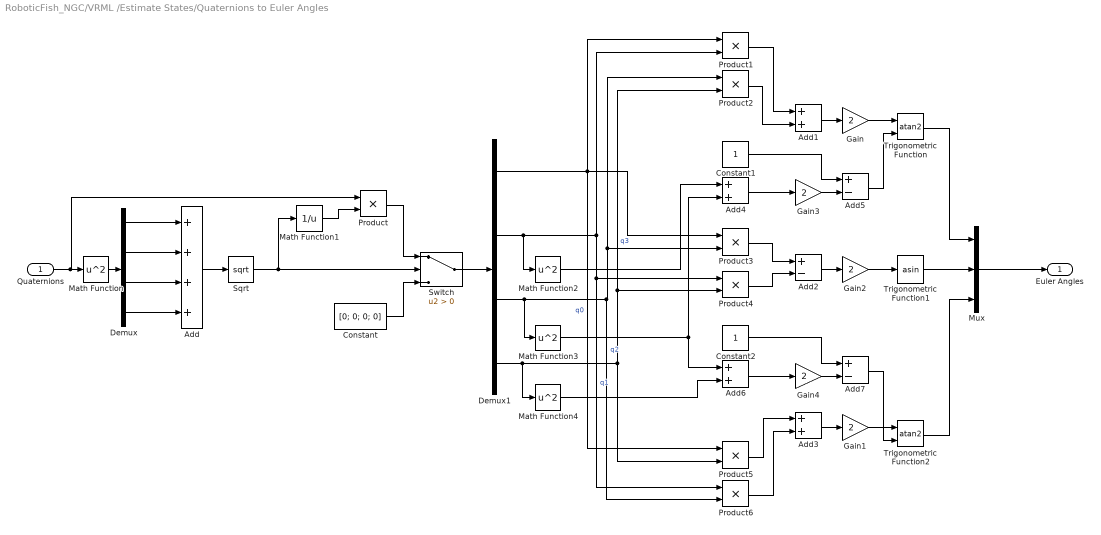
== system RoboticFish_NGC/VRML /Estimate States/Quaternions to Euler Angles ==
  Quaternions : Inport
  Add : Sum  Inputs=4
  Add{1,3..4,6} (4 alike) : Sum
  Add2 : Sum  Inputs=+-
  Add5 : Sum  Inputs=+-
  Add7 : Sum  Inputs=+-
  Constant : Constant  Value=[0; 0; 0; 0]
  Constant1 : Constant
  Constant2 : Constant
  Demux : Demux
  Demux1 : Demux
  Gain{,1..4} (5 alike) : Gain  Gain=2
  Math Function{,2..4} (4 alike) : Math  Operator=square  SignedPower=on
  Math Function1 : Math  Operator=reciprocal  SignedPower=on
  Mux : Mux  Inputs=3
  Product{,1..6} (7 alike) : Product
  Sqrt : Sqrt
  Switch : Switch  Criteria=u2 > Threshold  SaturateOnIntegerOverflow=off  InputSameDT=off
  Trigonometric Function : Trigonometry  Operator=atan2
  Trigonometric Function1 : Trigonometry  Operator=asin
  Trigonometric Function2 : Trigonometry  Operator=atan2
  Euler Angles : Outport  VectorParamsAs1DForOutWhenUnconnected=off
  wires:
  Quaternions/1 -> Product/1, Math Function/1
  Add/1 -> Sqrt/1
  Sqrt/1 -> Math Function1/1, Switch/2
  Constant/1 -> Switch/3
  Math Function1/1 -> Product/2
  Product/1 -> Switch/1
  Switch/1 -> Demux1/1
  Demux1/1 -> Product5/1, Product3/1, Product1/1  "q0"
  Demux1/2 -> Product6/1, Product4/1, Product1/2, Math Function2/1  "q1"
  Demux1/3 -> Product6/2, Product3/2, Product2/1, Math Function3/1  "q2"
  Demux1/4 -> Product5/2, Product4/2, Product2/2, Math Function4/1  "q3"
  Trigonometric Function1/1 -> Mux/2
  Mux/1 -> Euler Angles/1
  Trigonometric Function/1 -> Mux/1
  Trigonometric Function2/1 -> Mux/3
  Gain/1 -> Trigonometric Function/1
  Gain1/1 -> Trigonometric Function2/1
  Gain2/1 -> Trigonometric Function1/1
  Add1/1 -> Gain/1
  Add2/1 -> Gain2/1
  Add3/1 -> Gain1/1
  Product3/1 -> Add2/1
  Product4/1 -> Add2/2
  Product5/1 -> Add3/1
  Product6/1 -> Add3/2
  Product2/1 -> Add1/2
  Product1/1 -> Add1/1
  Add4/1 -> Gain3/1
  Gain3/1 -> Add5/2
  Constant1/1 -> Add5/1
  Add5/1 -> Trigonometric Function/2
  Add7/1 -> Trigonometric Function2/2
  Add6/1 -> Gain4/1
  Gain4/1 -> Add7/2
  Constant2/1 -> Add7/1
  Math Function2/1 -> Add4/1
  Math Function3/1 -> Add6/1, Add4/2
  Math Function4/1 -> Add6/2
  Demux/1 -> Add/1
  Demux/2 -> Add/2
  Demux/3 -> Add/3
  Demux/4 -> Add/4
  Math Function/1 -> Demux/1
